simulink model "test_zad_odwr"  (R2015b)
settings: Solver=VariableStepAuto  StartTime=0.0  StopTime=10.0  RelTol=1e-3
settings Model: Creator=lukinowy  LastModifiedBy=lukas

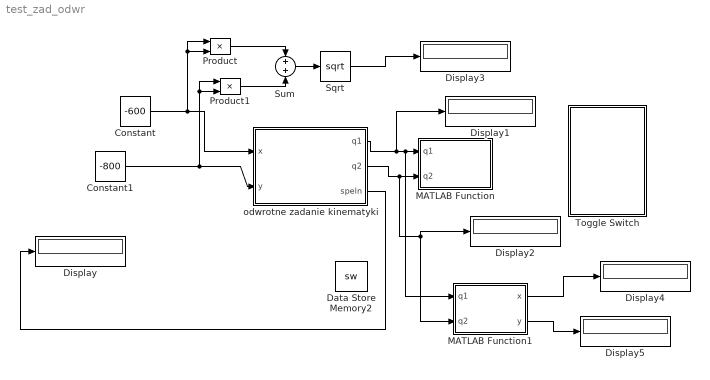
== system test_zad_odwr ==
  Constant : Constant  Value=-600
  Constant1 : Constant  Value=-800
  Data Store Memory2 : DataStoreMemory  DataStoreName=sw  ReadBeforeWriteMsg=warning  WriteAfterWriteMsg=warning  WriteAfterReadMsg=warning  InitialValue=1
  Display{,1..5} (6 alike) : Display
  MATLAB Function : MATLAB Function  TreatAsAtomicUnit=on
  MATLAB Function1 : MATLAB Function  TreatAsAtomicUnit=on
  Product : Product
  Product1 : Product
  Sqrt : Sqrt  SaturateOnIntegerOverflow=on
  Sum : Sum  Inputs=+|+
  Toggle Switch : Subsystem  DialogController=hmiCreateDDGDialog  IsWebBlock=on  mask(MWDashboardBlock){webBlockId=e4d935e1-5e3d-48c9-8083-7ccfc6df201e, webBlockType=toggleswitch, ShowInLibBrowser=on, ShowInitialText=on, HMISrcModelName=test_zad_odwr}
      mask prompts: webBlockId "WebBlock Id"; webBlockType "WebBlock Type"; HMISrcModelName "Source Model"
      mask Help: helpview([docroot '/mapfiles/simulink.map'], 'hmi_toggle_switch')
      mask Display:
      | if strcmp(get_param(bdroot(gcb),'BlockDiagramType'), 'library')
      |     image([(matlabroot) '/toolbox/simulink/hmi/icons/ToggleSwitch.png']);
      | end
  odwrotne zadanie kinematyki : MATLAB Function  TreatAsAtomicUnit=on
  wires:
  odwrotne zadanie kinematyki/1(q1) -> Display1/1, MATLAB Function1/1(q1), MATLAB Function/1(q1)
  odwrotne zadanie kinematyki/2(q2) -> MATLAB Function1/2(q2), Display2/1, MATLAB Function/2(q2)
  odwrotne zadanie kinematyki/3(speln) -> Display/1
  Constant/1 -> Product/2, Product/1, odwrotne zadanie kinematyki/1(x)
  Constant1/1 -> odwrotne zadanie kinematyki/2(y), Product1/1, Product1/2
  Product/1 -> Sum/1
  Product1/1 -> Sum/2
  Sum/1 -> Sqrt/1
  Sqrt/1 -> Display3/1
  MATLAB Function1/2(y) -> Display5/1
  MATLAB Function1/1(x) -> Display4/1

== system test_zad_odwr/Toggle Switch ==

== matlab function test_zad_odwr/MATLAB Function ==
  data: q1 input; q2 input
function fcn(q1,q2)
q1 = q1*pi/180;
q2 = q2*pi/180;

R1 = 630;
R2 = 510;
x1 = R1*cos(q1);
y1 = R1*sin(q1);
x2 = R1*cos(q1) - R2*cos(q2 - q1);
y2 = R1*sin(q1) + R2*sin(q2 - q1);
% x1 
% x2 
% y1 
% y2
figure(1)
plot([0 x1 x2],[0 y1 y2],'-*')
axis equal

== matlab function test_zad_odwr/odwrotne zadanie kinematyki ==
  data: x input; y input; q1 output; q2 output; speln output
function [q1,q2,speln] = fcn(x,y)
%#codegen
% Bierze po uwagę pomiar drugiego enkodera przy ustawianiu końcówki na oś y
% oś y linia bazowania, x - q1 i q2 odchylają się w kierunku x przy
% wychodzeniu z bazy
% R1 R2 [mm]
R1 = 630;
R2 = 510;
R = sqrt(x.^2 + y.^2);
if 0
    if R^2<(R1+R2)^2 && R^2 > (R1-R2)^2
        speln = 1;
        L = (R1.^2 + R2.^2 - R.^2)./(2*R1*R2);
        q2 = atan(sqrt(1-L^2)/L);

        if y<0
            q2=-abs(q2);
        else
            q2=abs(q2);
        end
        if R^2>R1^2+R2^2
            if q2>0
                q2=-q2+pi;
            else q2 = -q2 - pi; 
            end
        end
        q1 = atan2(y,x) - atan(R2*sin(q2)/(R1-R2*cos(q2)));
        q1 = q1*180/pi;
        q2 = q2*180/pi;
    else
        speln=0;
        q1=200;
        q2=200;
    end
elseif 1
    if R^2<(R1+R2)^2 && R^2 > (R1-R2)^2
        speln=1;
        L = (R1.^2 + R2.^2 - R.^2)./(2*R1*R2);
        q2 = atan2(sqrt(1-L^2),L);
        q1 = atan2(y,x) - atan(R2*sin(q2)/(R1-R2*cos(q2)));
        q1 = q1*180/pi;
        q2 = q2*180/pi;
        if q1<-180
            q1=q1+360;
        elseif q1>180
            q1=q1-360;
        end
        if q2<-180
            q2=q2+360;
        elseif q2>180
            q2=q2-360;
        end
    else
        q1 = 200;
        q2 = 200;
        speln=0;
    end
end

== matlab function test_zad_odwr/MATLAB Function1 ==
  data: x output; q1 input; y output; q2 input
function [x,y] = fcn(q1,q2)
%#codegen
q1 = pi/180*q1;
q2 = pi/180*q2;
R1 = 630;
R2 = 510;
y = R1*sin(q1)+R2*sin(q2-q1);
x = R1*cos(q1)-R2*cos(q2-q1);
